simulink model "uGrid_1PH_hd_caso3"  (R2017a)
settings: Solver=VariableStepAuto  StartTime=0.0  StopTime=5  FixedStep=1e-6  MaxStep=1e-4  RelTol=1e-3
PreLoadFcn:
  | SimulinkInit
InitFcn:
  | SimulinkInit
StartFcn:
  | SimulinkInit
StopFcn:
  | EndingScript
undefined symbols (not defined in the file or in its folder): G, GF, Ion, J, K1, K2, K3, Lithium, P, Tao1, Tao2
libraries: powerlib x60, truetime x17, dsparch4 x12, powerlib_meascontrol x4, electricdrivelib x1, simulink x1
(part 1 of 2)
settings Model: SimulationMode=accelerator  Creator=erich  LastModifiedBy=carma

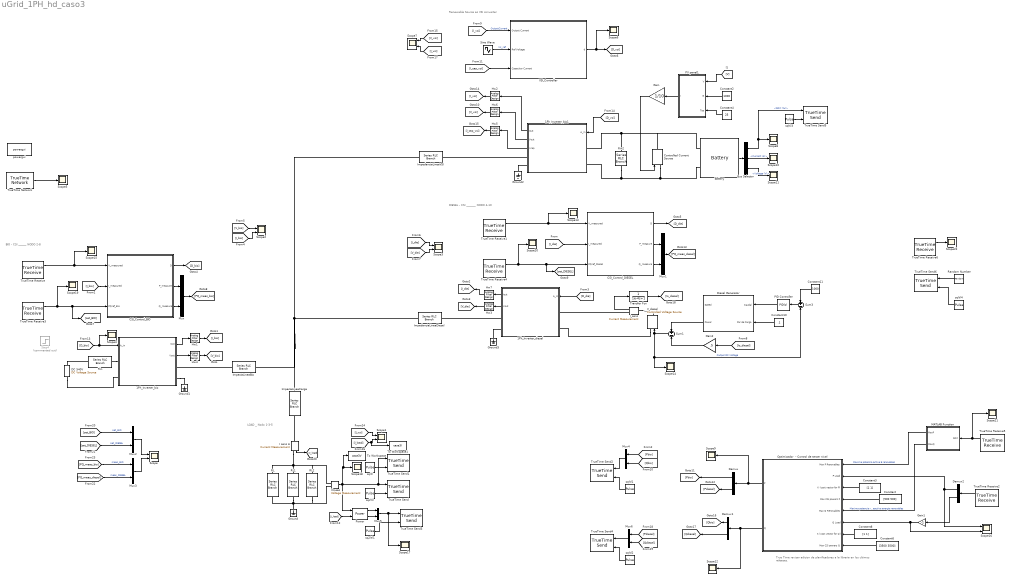
== system uGrid_1PH_hd_caso3 ==
  note: True Time revisar adicion de planificadores
      | a la libreria en los ultimos releases.
  note: Renewable Source as VSI converter
  note: LOAD _ Nodo 1-3-5
  note: BIO - CSI ______ NODO 2-8
  note: DIESEL - CSI _______ NODO 4-10
  1Ph_Inverter_bio : Subsystem  mask{st_time=4, f_sw=12000, samp_f=1e-6}
      mask prompts: st_time "Tiempo muerto (Start)"; f_sw "Switching frequency"; samp_f "samplig"
      mask Display:
      | port_label('input', 1, 'd', 'texmode', 'on')
      | 
      | port_label('lconn', 1, 'DC +')
      | port_label('lconn', 2, 'DC -')
      | 
      | 
      | port_label('rconn', 1, 'V_{out+}')
      | port_label('rconn', 2, 'B_{out-}')
      | 
      | 
      | port_label('output', 1, 'I_{out}', 'texmode', 'on')
      | port_label('output', 2, 'V_{out}', 'texmode', 'on')
      | 
      | plot([0.1 .9], [0.1 .9])
      | plot([0.2 .4], [.7 .7])
      | plot([0.2 .24], [.65 .65])
      | plot([0.28 .32], [.65 .65])
      | plot([0.36 .40], [.65 .65])
      | 
      | plot([.5:.01:.7], .25+sin(30*[.2:.01:.4])/10)
  1Ph_Inverter_bio1 : Subsystem  mask{st_time=1e-3, f_sw=12000, samp_f=1e-6}
      mask prompts: st_time "Tiempo muerto (Start)"; f_sw "Switching frequency"; samp_f "samplig"
      mask Display:
      | port_label('input', 1, 'd', 'texmode', 'on')
      | 
      | port_label('lconn', 1, 'DC +')
      | port_label('lconn', 2, 'DC -')
      | 
      | 
      | port_label('rconn', 1, 'V_{out+}')
      | port_label('rconn', 2, 'B_{out-}')
      | 
      | 
      | port_label('output', 1, 'I_{out}', 'texmode', 'on')
      | port_label('output', 2, 'V_{out}', 'texmode', 'on')
      | port_label('output', 3, 'I_{cap}', 'texmode', 'on')
      | 
      | plot([0.1 .9], [0.1 .9])
      | plot([0.2 .4], [.7 .7])
      | plot([0.2 .24], [.65 .65])
      | plot([0.28 .32], [.65 .65])
      | plot([0.36 .40], [.65 .65])
      | 
      | plot([.5:.01:.7], .25+sin(30*[.2:.01:.4])/10)
  1Ph_Inverter_diesel : Subsystem  mask{st_time=4, f_sw=12000, samp_f=1e-6}
      mask prompts: st_time "Tiempo muerto (Start)"; f_sw "Switching frequency"; samp_f "Sampling frequency"
      mask Display:
      | port_label('input', 1, 'd', 'texmode', 'on')
      | 
      | port_label('lconn', 1, 'DC +')
      | port_label('lconn', 2, 'DC -')
      | 
      | 
      | port_label('rconn', 1, 'V_{out+}')
      | port_label('rconn', 2, 'B_{out-}')
      | 
      | 
      | port_label('output', 1, 'I_{out}', 'texmode', 'on')
      | port_label('output', 2, 'V_{out}', 'texmode', 'on')
      | 
      | plot([0.1 .9], [0.1 .9])
      | plot([0.2 .4], [.7 .7])
      | plot([0.2 .24], [.65 .65])
      | plot([0.28 .32], [.65 .65])
      | plot([0.36 .40], [.65 .65])
      | 
      | plot([.5:.01:.7], .25+sin(30*[.2:.01:.4])/10)
  Battery : electricdrivelib/Extra Sources/Battery  BatType=Lithium-Ion  ShowTempParam=off  ThermalPreset=no  ShowAgeParam=off  NomV=1100  NomQ=.5  SOC=100  Batt_Tr=10e-3  PresetModel=off  MaxQ=1  MinV=825  FullV=1280.3859  Dis_rate=200  R=50e-3  Normal_OP=0.90435  expZone="[1188.4244    0.049130435]"  current=[6.5 13 32.5 50]  Units=Time  Tci=20  NomT=20  T2=-30  MaxQ2=4.8  FullV2=7.1  Normal_OP2=5.655  expZone2="[6.58           1]"  Rca=0.6  ti=2000  Dp=0  Neq0=0  Tsim=1e6  Ta1=25  Qeol=5.4*0.9  Reol=0.013333*1.2  Char_age=[2.3478, 3]  Dis_age=[2.3478, 10]  N1=1500  N2=10500  N3=1000  N4=1400  Ta2=45  N5=950
  Bus Selector : BusSelector  OutputSignals=SOC (%),Current (A),Voltage (V)
  CSI_Control_BIO : Subsystem
  CSI_Control_DIESEL : Subsystem
  Constant : Constant  Value=[500 500]
  Constant10 : Constant  Value=.1
  Constant11 : Constant  Value=1000
  Constant2 : Constant  Value=1000
  Constant3 : Constant  Value=[1 1]
  Constant4 : Constant  Value=25
  Constant6 : Constant  Value=[3500 3500]
  Constant8 : Constant  Value=[1 1]
  Controlled Current Source : powerlib/Electrical Sources/Controlled Current Source  Initialize=on  Source_Type=AC  Amplitude=0  Phase=0  Frequency=0  Measurements=None
  DC 540V : powerlib/Electrical Sources/DC Voltage Source  Amplitude=1000  Measurements=None
  Demux : Demux  Outputs=2
  Demux1 : Demux  Outputs=2
  Demux2 : Demux  Outputs=2
  Diesel Generator : Subsystem
  Gain : Gain  Gain=1/10
  Gain1 : Gain  Gain=-1
  Gain2 : Gain  Gain=.5
  Ground{,1..3} (4 alike) : powerlib/Elements/Ground  LConnTagsString=a
  Hw{1..7} (7 alike) : dsparch4/Analog Filter Design  method=Bessel  filttype=Lowpass  N=2  Wlo=7000*2*pi  Whi=80  Rp=2  Rs=80
  I sens A : powerlib/Measurements/Current Measurement  PhasorSimulation=off  OutputType=Complex  PSBequivalent=0
  I_sens : powerlib/Measurements/Current Measurement  PhasorSimulation=off  OutputType=Complex  PSBequivalent=0
  ImpeciaLineaBio : powerlib/Elements/Series RLC Branch  LConnTagsString=__new0  RConnTagsString=__new0  BranchType=RL  Resistance=.01  Inductance=1e-6  SetiL0=off  InitialCurrent=0  Capacitance=1e-6  Setx0=off  InitialVoltage=0  Measurements=None
  ImpeciaLineaCarga : powerlib/Elements/Series RLC Branch  LConnTagsString=__new0  RConnTagsString=__new0  BranchType=RL  Resistance=.01  Inductance=1e-6  SetiL0=off  InitialCurrent=0  Capacitance=1e-6  Setx0=off  InitialVoltage=0  Measurements=None
  ImpedanciaLineaDiesel : powerlib/Elements/Series RLC Branch  LConnTagsString=__new0  RConnTagsString=__new0  BranchType=RL  Resistance=.01  Inductance=1e-6  SetiL0=off  InitialCurrent=0  Capacitance=1e-6  Setx0=off  InitialVoltage=0  Measurements=None
  ImpedanciaLineaVSI : powerlib/Elements/Series RLC Branch  LConnTagsString=__new0  RConnTagsString=__new0  BranchType=R  Resistance=.01  Inductance=1e-6  SetiL0=off  InitialCurrent=0  Capacitance=1e-6  Setx0=off  InitialVoltage=0  Measurements=None
  MATLAB Function : MATLAB Function  TreatAsAtomicUnit=on
  Mux{,1..6} (7 alike) : Mux  Inputs=2
  Optimizador  - Control de tercer nivel : Subsystem
  PID Controller : simulink/Continuous/PID Controller  Controller=PID  TimeDomain=Continuous-time  SampleTime=-1  IntegratorMethod=Forward Euler  FilterMethod=Forward Euler  Form=Parallel  UseFilter=on  ControllerParametersSource=internal  P=0.000853612192208084  I=3.94394231511782e-05  D=0.00224356290205903  N=0.155980576752107  InitialConditionSource=internal  InitialConditionForIntegrator=0  InitialConditionForFilter=0  ExternalReset=none  LimitOutput=off  UpperSaturationLimit=inf  LowerSaturationLimit=-inf  LinearizeAsGain=on  AntiWindupMode=none  Kb=1  TrackingMode=off  Kt=1  PParamMin=[]  PParamMax=[]  IParamMin=[]  IParamMax=[]  DParamMin=[]  DParamMax=[]  NParamMin=[]  NParamMax=[]  KbParamMin=[]  KbParamMax=[]  KtParamMin=[]  KtParamMax=[]  POutMin=[]  POutMax=[]  IOutMin=[]  IOutMax=[]  DOutMin=[]  DOutMax=[]  NOutMin=[]  NOutMax=[]  KbOutMin=[]  KbOutMax=[]  KtOutMin=[]  KtOutMax=[]  IntegratorOutMin=[]  IntegratorOutMax=[]  FilterOutMin=[]  FilterOutMax=[]  SumOutMin=[]  SumOutMax=[]  SumI1OutMin=[]  SumI1OutMax=[]  SumI2OutMin=[]  SumI2OutMax=[]  SumI3OutMin=[]  SumI3OutMax=[]  SumDOutMin=[]  SumDOutMax=[]  SaturationOutMin=[]  SaturationOutMax=[]  IntegratorContinuousStateAttributes=''  IntegratorStateMustResolveToSignalObject=off  IntegratorRTWStateStorageClass=Auto  FilterContinuousStateAttributes=''  FilterStateMustResolveToSignalObject=off  FilterRTWStateStorageClass=Auto  DifferentiatorICPrevScaledInput=0  DifferentiatorOutMin=[]  DifferentiatorOutMax=[]  InitialConditionSetting=State (most efficient)
  PV panel1 : Subsystem
      mask Display: image('panel.jpg')
  Power : powerlib_meascontrol/Measurements/Power  Freq=60  Vinit=[1, 0]  Iinit=[1, 0]  Ts=0
      settings: SourceProductName=Simscape Power Systems
  RL : powerlib/Elements/Series RLC Branch  LConnTagsString=__new0  RConnTagsString=__new0  BranchType=R  Resistance=10  Inductance=500e-3  SetiL0=off  InitialCurrent=0  Capacitance=100e-6  Setx0=off  InitialVoltage=0  Measurements=None
  RL1 : powerlib/Elements/Series RLC Branch  LConnTagsString=__new0  RConnTagsString=__new0  BranchType=RL  Resistance=10  Inductance=5.2  SetiL0=off  InitialCurrent=0  Capacitance=100e-6  Setx0=off  InitialVoltage=0  Measurements=None
  RL2 : powerlib/Elements/Series RLC Branch  LConnTagsString=__new0  RConnTagsString=__new0  BranchType=C  Resistance=30  Inductance=500e-3  SetiL0=off  InitialCurrent=0  Capacitance=2000e-6  Setx0=off  InitialVoltage=0  Measurements=None
  Random Number : RandomNumber  SampleTime=0.1
  Rin : powerlib/Elements/Series RLC Branch  LConnTagsString=__new0  RConnTagsString=__new0  BranchType=R  Resistance=.001  Inductance=0  SetiL0=off  InitialCurrent=0  Capacitance=0  Setx0=off  InitialVoltage=0  Measurements=None
  Rin2 : powerlib/Elements/Series RLC Branch  LConnTagsString=__new0  RConnTagsString=__new0  BranchType=C  Resistance=.001  Inductance=0  SetiL0=off  InitialCurrent=0  Capacitance=1000e-6  Setx0=off  InitialVoltage=0  Measurements=None
  Scope{,1..3,7,16} (6 alike) : Scope  NumInputPorts=2
  Scope{4..6,8..15,17..22} (17 alike) : Scope
  Sine Wave : Sin  Amplitude=170  Frequency=2*pi*60  SampleTime=0
  Step4 : Step  Commented=on  Time=[2.3 2.3]  Before=[0 0]  After=[500 3500]  SampleTime=0
  Sum1 : Sum  Inputs=+-
  Sum3 : Sum  Inputs=+-
  To Workspace : ToWorkspace  VariableName=case3V  SaveFormat=Timeseries  SampleTime=1e-4
  To Workspace1 : ToWorkspace  VariableName=case3I  SaveFormat=Timeseries  SampleTime=1e-4
  Transfer Fcn : TransferFcn  Denominator=[1e-4 1]
  TrueTime Network : truetime/TrueTime Network  nwtype=CSMA/CD (Ethernet)  nwnbr=1  nnodes=14  rate=1000e7  minsize=100  lossprob=0  seed=0  bandwidths=[0.5 0.5]  slotsize=512  schedule=[1 1 2]  memsize=80000  buftype=Common buffer  overflow=Retransmit  dynSchedule=0  miniSlotSize=0  NIT=0  QSortMode=FIFO  sync=0  irtSchedule=0  nrtLength=0  nodeGraph=0  scheduleoutput=on
  TrueTime Receive : truetime/TrueTime Receive  nwnbr=1  receiver=2  outdim=1  triggeroutput=on  senderoutput=off  lengthoutput=off  priorityoutput=off  timestampoutput=off  signalpoweroutput=off  msgIDoutput=off
  TrueTime Receive1 : truetime/TrueTime Receive  nwnbr=1  receiver=4  outdim=1  triggeroutput=on  senderoutput=off  lengthoutput=off  priorityoutput=off  timestampoutput=off  signalpoweroutput=off  msgIDoutput=off
  TrueTime Receive2 : truetime/TrueTime Receive  nwnbr=1  receiver=6  outdim=2  triggeroutput=on  senderoutput=off  lengthoutput=off  priorityoutput=off  timestampoutput=off  signalpoweroutput=off  msgIDoutput=off
  TrueTime Receive3 : truetime/TrueTime Receive  nwnbr=1  receiver=8  outdim=2  triggeroutput=on  senderoutput=off  lengthoutput=off  priorityoutput=off  timestampoutput=off  signalpoweroutput=off  msgIDoutput=off
  TrueTime Receive4 : truetime/TrueTime Receive  nwnbr=1  receiver=10  outdim=2  triggeroutput=on  senderoutput=off  lengthoutput=off  priorityoutput=off  timestampoutput=off  signalpoweroutput=off  msgIDoutput=off
  TrueTime Receive5 : truetime/TrueTime Receive  nwnbr=1  receiver=12  outdim=1  triggeroutput=on  senderoutput=off  lengthoutput=off  priorityoutput=off  timestampoutput=off  signalpoweroutput=off  msgIDoutput=off
  TrueTime Receive6 : truetime/TrueTime Receive  nwnbr=1  receiver=14  outdim=1  triggeroutput=on  senderoutput=off  lengthoutput=off  priorityoutput=off  timestampoutput=off  signalpoweroutput=off  msgIDoutput=off
  TrueTime Send : truetime/TrueTime Send  trigger=falling  nwnbr=1  sender=3  indim=1  recsource=internal  receiver=4  lengthsource=internal  length=16  priosource=internal  prio=1  msgIDsource=internal  msgID=1  dynamicSegment=dynamic
  TrueTime Send1 : truetime/TrueTime Send  trigger=falling  nwnbr=1  sender=1  indim=1  recsource=internal  receiver=2  lengthsource=internal  length=16  priosource=internal  prio=1  msgIDsource=internal  msgID=0  dynamicSegment=dynamic
  TrueTime Send2 : truetime/TrueTime Send  trigger=falling  nwnbr=1  sender=7  indim=2  recsource=internal  receiver=8  lengthsource=internal  length=16  priosource=internal  prio=1  msgIDsource=internal  msgID=0  dynamicSegment=dynamic
  TrueTime Send3 : truetime/TrueTime Send  trigger=falling  nwnbr=1  sender=5  indim=2  recsource=internal  receiver=6  lengthsource=internal  length=16  priosource=internal  prio=1  msgIDsource=internal  msgID=0  dynamicSegment=dynamic
  TrueTime Send4 : truetime/TrueTime Send  trigger=falling  nwnbr=1  sender=9  indim=2  recsource=internal  receiver=10  lengthsource=internal  length=16  priosource=internal  prio=1  msgIDsource=internal  msgID=0  dynamicSegment=dynamic
  TrueTime Send5 : truetime/TrueTime Send  trigger=falling  nwnbr=1  sender=11  indim=1  recsource=internal  receiver=12  lengthsource=internal  length=16  priosource=internal  prio=1  msgIDsource=internal  msgID=0  dynamicSegment=dynamic
  TrueTime Send6 : truetime/TrueTime Send  trigger=falling  nwnbr=1  sender=13  indim=1  recsource=internal  receiver=14  lengthsource=internal  length=16384*16  priosource=internal  prio=1  msgIDsource=internal  msgID=0  dynamicSegment=dynamic
  VSI_Controller : Subsystem
  V_diesel : powerlib/Electrical Sources/Controlled Voltage Source  Initialize=on  Source_Type=AC  Amplitude=0  Phase=0  Frequency=0  Measurements=None
  Vmeas : powerlib/Measurements/Voltage Measurement  PhasorSimulation=off  OutputType=Complex  PSBequivalent=0
  powergui : powerlib/powergui  Priority=1  SimulationMode=Continuous  SampleTime=50e-6  frequency=60  Iterations=50  frequencyindice=0  Pbase=100e6  ErrMax=1e-4  UnitsV=kV  UnitsW=MW  buscounter=0  FunctionMessages=off  echomessages=off  EnableUseOfTLC=off  CurrentSourceSwitches=off  DisableSnubberDevices=off  DisableRonSwitches=off  DisableVfSwitches=off  DisplayEquations=off  SolverType=Tustin/Backward Euler (TBE)  Interpol=off  ExternalGateDelay=off  methode=off  Ts=100  x0status=blocks  SPID=on  SwTol=0  HookPort=off  RestoreLinks=warning  ResistiveCurrentMeasurement=off  Frange=[0:2:500]  Ylog=off  Xlog=on  ShowGrid=off  save=off  variable=ZData  structure=0  ZoomFFT=off  StartTime=0.0  cycles=1  DisplayStyle=1  fundamental=60  FreqAxis=off  MaxFrequency=1000  frequencyindicesteady=1  RmsSteady=1  display=off
  sq(t) : DiscretePulseGenerator  PulseType=Time based  Period=1e-4  PhaseDelay=1e-3
  sq(t)1 : DiscretePulseGenerator  PulseType=Time based  Period=.5  PhaseDelay=2e-3
  sq(t)2 : DiscretePulseGenerator  PulseType=Time based  Period=.5  PhaseDelay=3e-3
  sq(t)3 : DiscretePulseGenerator  PulseType=Time based  Period=.05  PhaseDelay=2e-3
  sq(t)4 : DiscretePulseGenerator  PulseType=Time based  Period=.5e-5  PhaseDelay=7e-3
  sq2(t) : DiscretePulseGenerator  PulseType=Time based  Period=1e-4  PhaseDelay=5e-3
  sq2(t)1 : DiscretePulseGenerator  PulseType=Time based  Period=.05
  wires:
  [D_bio] -> Scope4/1, 1Ph_Inverter_bio/1(A_in)
  [D_die] -> 1Ph_Inverter_diesel/1(A_in)
  [I_bio] -> Scope2/2
  [V_bio] -> Scope2/1
  [I_die] -> Scope3/1
  [V_die] -> Scope3/2
  1Ph_Inverter_bio/2(Vout) -> Hw4/1
  1Ph_Inverter_bio/1(Iout) -> Hw1/1
  Hw1/1 -> [I_bio]
  Hw4/1 -> [V_bio]
  1Ph_Inverter_diesel/1(Iout) -> Hw7/1
  Hw7/1 -> [I_die]
  Hw3/1 -> [V_die]
  1Ph_Inverter_diesel/2(Vout) -> Hw3/1
  I sens A/1 -> [I_load]
  CSI_Control_BIO/1(D) -> [D_bio]
  [I_bio] -> CSI_Control_BIO/2(I_measured)
  TrueTime Receive/1 -> Scope15/1, CSI_Control_BIO/1(V_measured)
  CSI_Control_DIESEL/1(D) -> [D_die]
  [I_die] -> CSI_Control_DIESEL/2(I_measured)
  TrueTime Receive1/1 -> Scope13/1, CSI_Control_DIESEL/1(V_measured)
  [I_vsi] -> Scope1/1
  [I_load] -> To Workspace1/1, Scope1/2
  Mux/1 -> [PQ_meas_bio]
  Mux1/1 -> [PQ_meas_diesel]
  [set_DIESEL] -> Mux2/2  "set_DIESEL"
  [set_BIO] -> Mux2/1  "set_BIO"
  Mux2/1 -> Scope/1
  Mux3/1 -> Scope/2
  [PQ_meas_diesel] -> Mux3/2  "meas_DIESEL"
  [PQ_meas_bio] -> Mux3/1  "meas_BIO"
  CSI_Control_BIO/2(P_measure) -> Mux/1
  CSI_Control_BIO/3(Q_measure) -> Mux/2
  CSI_Control_DIESEL/2(P_measure) -> Mux1/1
  CSI_Control_DIESEL/3(Q_measure) -> Mux1/2
  VSI_Controller/1(d) -> Scope6/1, [D_vsi]
  [I_vsi] -> VSI_Controller/1(Output Current)  "OutputCurrent"
  Sine Wave/1 -> VSI_Controller/2(Ref Voltage)  "Vc_ref"
  [I_cap_vsi] -> VSI_Controller/3(Capacitor Current)
  Hw5/1 -> [I_cap_vsi]
  1Ph_Inverter_bio1/3(I cap) -> Hw5/1
  1Ph_Inverter_bio1/2(Vout) -> Hw6/1
  1Ph_Inverter_bio1/1(Iout) -> Hw2/1
  [D_vsi] -> 1Ph_Inverter_bio1/1(A_in)
  Hw6/1 -> [V_vsi]
  Hw2/1 -> [I_vsi]
  [V_vsi] -> Scope7/1
  [I_vsi] -> Scope7/2
  Bus Selector/1 -> TrueTime Send5/1, Scope8/1  "<SOC (%)>"
  Bus Selector/3 -> Scope11/1  "<Voltage (V)>"
  Bus Selector/2 -> Scope10/1  "<Current (A)>"
  Battery/1 -> Bus Selector/1
  Constant2/1 -> PV panel1/2(G)
  [V] -> PV panel1/1(V)
  Constant4/1 -> PV panel1/3(Top)
  PV panel1/1(I) -> Gain/1
  Gain/1 -> Controlled Current Source/1
  TrueTime Receive4/1 -> Scope20/1, [set_DIESEL], CSI_Control_DIESEL/3(PQref_Diesel)
  Vmeas/1 -> To Workspace/1, Scope18/1, Power/1, TrueTime Send1/1, TrueTime Send/1
  sq2(t)/1 -> TrueTime Send/2
  TrueTime Network/1 -> Scope5/1
  MATLAB Function/1(MaxP) -> Optimizador  - Control de tercer nivel/1(Max P Renovables)  "Maxima potencia activa E renovables"
  Demux2/1 -> Optimizador  - Control de tercer nivel/2(P Load), Scope16/1
  Constant3/1 -> Optimizador  - Control de tercer nivel/3(K (cost vector for P))
  Constant/1 -> Optimizador  - Control de tercer nivel/4(Max CSI powers P)
  MATLAB Function/2(MaxQ) -> Optimizador  - Control de tercer nivel/5(Max Q Renovables)  "Maxima potencia reactiva energia renovables"
  Demux2/2 -> Gain1/1
  Constant8/1 -> Optimizador  - Control de tercer nivel/7(K (cost vector for Q))
  Constant6/1 -> Optimizador  - Control de tercer nivel/8(Max CSI powers Q)
  Optimizador  - Control de tercer nivel/2(Q) -> Demux1/1, Scope12/1
  Optimizador  - Control de tercer nivel/1(P) -> Demux/1, Scope9/1
  Demux/1 -> [Pbio]
  Demux/2 -> [Pdiesel]
  Demux1/2 -> [Qdiesel]
  Demux1/1 -> [Qbio]
  Constant10/1 -> Diesel Generator/2(Par de Carga)
  sq(t)/1 -> TrueTime Send1/2
  Transfer Fcn/1 -> [Io_diesel]
  I_sens/1 -> Transfer Fcn/1
  Gain2/1 -> Sum1/2
  [Io_diesel] -> Gain2/1
  Constant11/1 -> Sum3/1
  Sum3/1 -> PID Controller/1
  Sum1/1 -> Scope14/1, Sum3/2, V_diesel/1  "Output DC Voltage"
  PID Controller/1 -> Diesel Generator/1(Caudal)
  Diesel Generator/2(Power) -> Sum1/1
  sq(t)1/1 -> TrueTime Send2/2
  [Qbio] -> Mux4/2
  [Pbio] -> Mux4/1
  Mux4/1 -> TrueTime Send2/1
  [I_load] -> Power/2
  Power/1 -> Mux5/1
  Power/2 -> Mux5/2
  Mux5/1 -> Scope17/1, TrueTime Send3/1
  sq2(t)1/1 -> TrueTime Send3/2
  TrueTime Receive2/1 -> Demux2/1
  [Pdiesel] -> Mux6/1
  [Qdiesel] -> Mux6/2
  Mux6/1 -> TrueTime Send4/1
  sq(t)2/1 -> TrueTime Send4/2
  TrueTime Receive3/1 -> Scope19/1, [set_BIO], CSI_Control_BIO/3(PQref_Bio)
  Gain1/1 -> Scope16/2, Optimizador  - Control de tercer nivel/6(Q Load)
  sq(t)3/1 -> TrueTime Send5/2
  TrueTime Receive5/1 -> Scope21/1, MATLAB Function/1(SOC)
  sq(t)4/1 -> TrueTime Send6/2
  Random Number/1 -> TrueTime Send6/1
  TrueTime Receive6/1 -> Scope22/1
  connections:
  RL/LConn1 -- RL2/LConn1 -- Vmeas/LConn1 -- I sens A/RConn1 -- RL1/LConn1
  Ground/LConn1 -- Vmeas/LConn2 -- RL2/RConn1 -- RL1/RConn1 -- RL/RConn1
  1Ph_Inverter_bio/RConn2 -- Ground1/LConn1
  DC 540V/LConn1 -- 1Ph_Inverter_bio/LConn2
  Rin/RConn1 -- 1Ph_Inverter_bio/LConn1
  1Ph_Inverter_diesel/RConn2 -- Ground3/LConn1
  1Ph_Inverter_diesel/RConn1 -- ImpedanciaLineaDiesel/RConn1
  DC 540V/RConn1 -- Rin/LConn1
  1Ph_Inverter_bio1/RConn2 -- Ground2/LConn1
  Rin2/RConn1 -- 1Ph_Inverter_bio1/LConn2 -- Controlled Current Source/LConn1 -- Battery/LConn2
  Rin2/LConn1 -- Controlled Current Source/RConn1 -- Battery/LConn1 -- 1Ph_Inverter_bio1/LConn1
  V_diesel/LConn1 -- 1Ph_Inverter_diesel/LConn2
  I_sens/LConn1 -- V_diesel/RConn1
  I_sens/RConn1 -- 1Ph_Inverter_diesel/LConn1
  ImpeciaLineaBio/LConn1 -- 1Ph_Inverter_bio/RConn1
  ImpedanciaLineaDiesel/LConn1 -- ImpedanciaLineaVSI/LConn1 -- ImpeciaLineaCarga/LConn1 -- ImpeciaLineaBio/RConn1
  1Ph_Inverter_bio1/RConn1 -- ImpedanciaLineaVSI/RConn1
  I sens A/LConn1 -- ImpeciaLineaCarga/RConn1

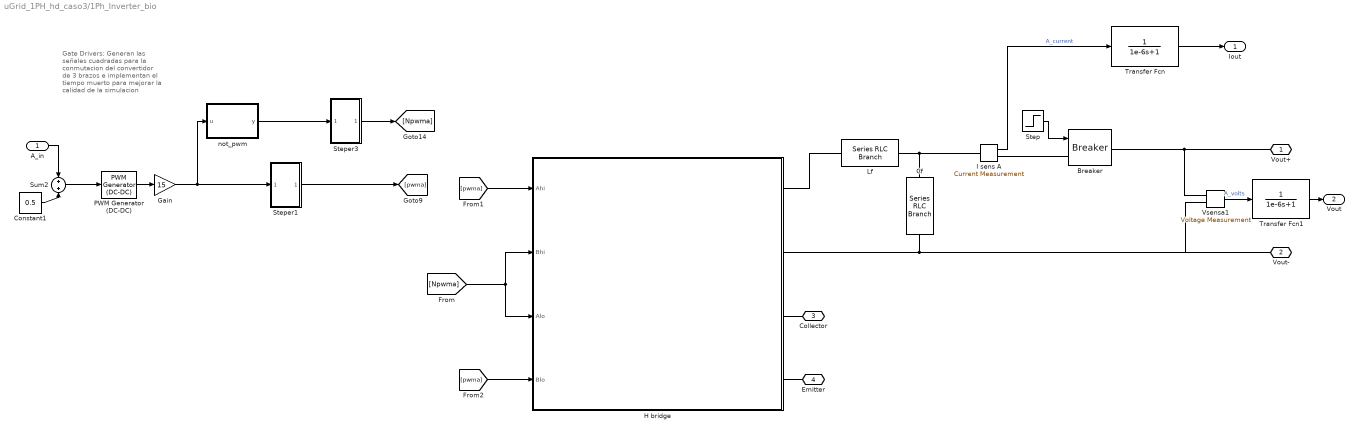
== system uGrid_1PH_hd_caso3/1Ph_Inverter_bio ==
  note: Gate Drivers: Generan las señales cuadradas para
      | la conmutacion del convertidor de 3 brazos e implementan el
      | tiempo muerto para mejorar la calidad de la simulacion
  A_in : Inport
  Breaker : powerlib/Elements/Breaker  InitialState=0  SwitchingTimes="[1/60  5/60]"  External=on  BreakerResistance=0.01  SnubberResistance=1e6  SnubberCapacitance=inf  Measurements=None  MoreParameters=on  NoBreakLoop=off
      settings: SourceProductName=Simscape Power Systems
  Cf : powerlib/Elements/Series RLC Branch  LConnTagsString=__new0  RConnTagsString=__new0  BranchType=C  Resistance=1  Inductance=1e-3  SetiL0=off  InitialCurrent=0  Capacitance=22e-6  Setx0=off  InitialVoltage=0  Measurements=None
  Constant1 : Constant  Value=0.5
  Gain : Gain  Gain=15
  H bridge : Subsystem
      mask Display:
      | port_label('input', 1, '\fontsize{12} Ahi', 'texmode', 'on')
      | port_label('input', 2, '\fontsize{12} Alo', 'texmode', 'on')
      | port_label('input', 3, '\fontsize{12} Bhi', 'texmode', 'on')
      | port_label('input', 4, '\fontsize{12} Blo', 'texmode', 'on')
      | 
      | 
      | port_label('rconn', 1, '\fontsize{12} V_{out} +', 'texmode', 'on')
      | port_label('rconn', 2, '\fontsize{12} V_{out} -', 'texmode', 'on')
      | 
      | port_label('rconn', 3, '\fontsize{12} Collector', 'texmode', 'on')
      | port_label('rconn', 4, '\fontsize{12} Emitter', 'texmode', 'on')
      | 
      | lvx = [.1 .1];
      | lvy = [.1 .2];
      | lhx = [.1 .2];
      | lhy = [.1 .1];
      | 
      | 
      | % se dibujan los interruptores de la izquierda
      | plot(lvx+.07, lvy*.8+.028+.1)
      | plot(lvx+.1, lvy+.1)
      | plot(lhx*.5+.15, lhy+.1)
      | plot(lhx*.5+.15, lhy+.2)
      | plot(lhx*.5+.07, lhy+.15)
      | 
      | d=0.5;
      | 
      | plot(lvx+.07, lvy*.8+.028+.1+d)
      | plot(lvx+.1, lvy+.1+d)
      | plot(lhx*.5+.15, lhy+.1+d)
      | plot(lhx*.5+.15, lhy+.2+d)
      | plot(lhx*.5+.07, lhy+.15+d)
      | 
      | 
      | % se dibujan los interruptores del medio
      | h=.3;
      | 
      | %plot(lvx+.07+h, lvy*.8+.028+.1)
      | %plot(lvx+.1+h, lvy+.1)
      | %plot(lhx*.5+.15+h, lhy+.1)
      | %plot(lhx*.5+.15+h, lhy+.2)
      | %plot(lhx*.5+.07+h, lhy+.15)
      | 
      | %plot(lvx+.07+h, lvy*.8+.028+.1+d)
      | %plot(lvx+.1+h, lvy+.1+d)
      | %plot(lhx*.5+.15+h, lhy+.1+d)
      | %plot(lhx*.5+.15+h, lhy+.2+d)
      | %plot(lhx*.5+.07+h, lhy+.15+d)
      | 
      | % se dibujan los interruptores de la derecha
      | h=.6
      | 
      | plot(lvx+.07+h, lvy*.8+.028+.1)
      | plot(lvx+.1+h, lvy+.1)
      | plot(lhx*.5+.15+h, lhy+.1)
      | plot(lhx*.5+.15+h, lhy+.2)
      | plot(lhx*.5+.07+h, lhy+.15)
      | 
      | plot(lvx+.07+h, lvy*.8+.028+.1+d)
      | plot(lvx+.1+h, lvy+.1+d)
      | plot(lhx*.5+.15+h, lhy+.1+d)
      | plot(lhx*.5+.15+h, lhy+.2+d)
      | plot(lhx*.5+.07+h, lhy+.15+d)
      | 
      | 
      | % se conectan los interruptores.
      | plot(lvx+.15, lvy*4-.1)
      | %plot(lvx+.15+.3, lvy*4-.1)
      | plot(lvx+.15+.6, lvy*4-.1)
      | 
      | 
      | plot(lvx+.15, lvy+.7)
      | %plot(lvx+.15+.3, lvy+.7)
      | plot(lvx+.15+.6, lvy+.7)
      | 
      | plot(lvx+.15, lvy)
      | %plot(lvx+.15+.3, lvy)
      | plot(lvx+.15+.6, lvy)
      | 
      | plot(lhx*6-.35, lhy)
      | plot(lhx*6-.35, lhy+.8)
      | 
      | % raul esteban alzate 313 515 86 11
  I sens A : powerlib/Measurements/Current Measurement  PhasorSimulation=off  OutputType=Complex  PSBequivalent=0
  Lf : powerlib/Elements/Series RLC Branch  LConnTagsString=__new0  RConnTagsString=__new0  BranchType=RL  Resistance=.1  Inductance=40e-3  SetiL0=off  InitialCurrent=0  Capacitance=1e-6  Setx0=off  InitialVoltage=0  Measurements=None
  PWM Generator (DC-DC) : powerlib_meascontrol/Pulse & Signal Generators/PWM Generator (DC-DC)  Fsw=f_sw  Ts=samp_f
  Step : Step  Time=st_time  SampleTime=0
  Steper1 : Subsystem
  Steper3 : Subsystem
  Sum2 : Sum
  Transfer Fcn : TransferFcn  Denominator=[1e-6 1]
  Transfer Fcn1 : TransferFcn  Denominator=[1e-6 1]
  Vsensa1 : powerlib/Measurements/Voltage Measurement  PhasorSimulation=off  OutputType=Complex  PSBequivalent=0
  not_pwm : MATLAB Function  TreatAsAtomicUnit=on
  Vout+ : PMIOPort  Port=1  Side=Right
  Vout- : PMIOPort  Port=2  Side=Right
  Collector : PMIOPort  Port=3  Side=Left
  Emitter : PMIOPort  Port=4  Side=Left
  Iout : Outport
  Vout : Outport  Port=2
  wires:
  not_pwm/1(y) -> Steper3/1(In1)
  Sum2/1 -> PWM Generator (DC-DC)/1
  PWM Generator (DC-DC)/1 -> Gain/1
  Constant1/1 -> Sum2/2
  A_in/1 -> Sum2/1
  Steper1/1(Out1) -> [pwma]
  Steper3/1(Out1) -> [Npwma]
  Gain/1 -> Steper1/1(In1), not_pwm/1(u)
  [pwma] -> H bridge/1(Ahi)
  [Npwma] -> H bridge/2(Bhi), H bridge/3(Alo)
  [pwma] -> H bridge/4(Blo)
  I sens A/1 -> Transfer Fcn/1  "A_current"
  Vsensa1/1 -> Transfer Fcn1/1  "A_volts"
  Transfer Fcn/1 -> Iout/1
  Transfer Fcn1/1 -> Vout/1
  Step/1 -> Breaker/1
  connections:
  H bridge/RConn3 -- Collector/RConn1
  H bridge/RConn4 -- Emitter/RConn1
  Lf/LConn1 -- H bridge/RConn1
  H bridge/RConn2 -- Vsensa1/LConn2 -- Vout-/RConn1 -- Cf/RConn1
  Breaker/LConn1 -- I sens A/RConn1
  Breaker/RConn1 -- Vout+/RConn1 -- Vsensa1/LConn1
  Cf/LConn1 -- I sens A/LConn1 -- Lf/RConn1

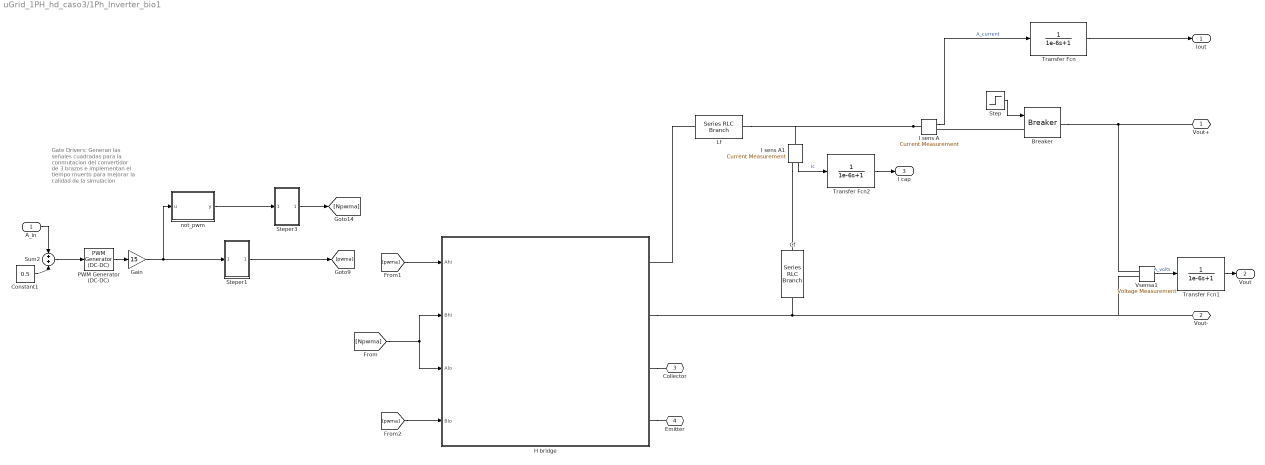
== system uGrid_1PH_hd_caso3/1Ph_Inverter_bio1 ==
  note: Gate Drivers: Generan las señales cuadradas para
      | la conmutacion del convertidor de 3 brazos e implementan el
      | tiempo muerto para mejorar la calidad de la simulacion
  A_in : Inport
  Breaker : powerlib/Elements/Breaker  InitialState=0  SwitchingTimes="[1/60  5/60]"  External=on  BreakerResistance=0.01  SnubberResistance=1e6  SnubberCapacitance=inf  Measurements=None  MoreParameters=on  NoBreakLoop=off
      settings: SourceProductName=Simscape Power Systems
  Cf : powerlib/Elements/Series RLC Branch  LConnTagsString=__new0  RConnTagsString=__new0  BranchType=C  Resistance=1  Inductance=1e-3  SetiL0=off  InitialCurrent=0  Capacitance=610e-6  Setx0=off  InitialVoltage=0  Measurements=None
  Constant1 : Constant  Value=0.5
  Gain : Gain  Gain=15
  H bridge : Subsystem
      mask Display:
      | port_label('input', 1, '\fontsize{12} Ahi', 'texmode', 'on')
      | port_label('input', 2, '\fontsize{12} Alo', 'texmode', 'on')
      | port_label('input', 3, '\fontsize{12} Bhi', 'texmode', 'on')
      | port_label('input', 4, '\fontsize{12} Blo', 'texmode', 'on')
      | 
      | 
      | port_label('rconn', 1, '\fontsize{12} V_{out} +', 'texmode', 'on')
      | port_label('rconn', 2, '\fontsize{12} V_{out} -', 'texmode', 'on')
      | 
      | port_label('rconn', 3, '\fontsize{12} Collector', 'texmode', 'on')
      | port_label('rconn', 4, '\fontsize{12} Emitter', 'texmode', 'on')
      | 
      | lvx = [.1 .1];
      | lvy = [.1 .2];
      | lhx = [.1 .2];
      | lhy = [.1 .1];
      | 
      | 
      | % se dibujan los interruptores de la izquierda
      | plot(lvx+.07, lvy*.8+.028+.1)
      | plot(lvx+.1, lvy+.1)
      | plot(lhx*.5+.15, lhy+.1)
      | plot(lhx*.5+.15, lhy+.2)
      | plot(lhx*.5+.07, lhy+.15)
      | 
      | d=0.5;
      | 
      | plot(lvx+.07, lvy*.8+.028+.1+d)
      | plot(lvx+.1, lvy+.1+d)
      | plot(lhx*.5+.15, lhy+.1+d)
      | plot(lhx*.5+.15, lhy+.2+d)
      | plot(lhx*.5+.07, lhy+.15+d)
      | 
      | 
      | % se dibujan los interruptores del medio
      | h=.3;
      | 
      | %plot(lvx+.07+h, lvy*.8+.028+.1)
      | %plot(lvx+.1+h, lvy+.1)
      | %plot(lhx*.5+.15+h, lhy+.1)
      | %plot(lhx*.5+.15+h, lhy+.2)
      | %plot(lhx*.5+.07+h, lhy+.15)
      | 
      | %plot(lvx+.07+h, lvy*.8+.028+.1+d)
      | %plot(lvx+.1+h, lvy+.1+d)
      | %plot(lhx*.5+.15+h, lhy+.1+d)
      | %plot(lhx*.5+.15+h, lhy+.2+d)
      | %plot(lhx*.5+.07+h, lhy+.15+d)
      | 
      | % se dibujan los interruptores de la derecha
      | h=.6
      | 
      | plot(lvx+.07+h, lvy*.8+.028+.1)
      | plot(lvx+.1+h, lvy+.1)
      | plot(lhx*.5+.15+h, lhy+.1)
      | plot(lhx*.5+.15+h, lhy+.2)
      | plot(lhx*.5+.07+h, lhy+.15)
      | 
      | plot(lvx+.07+h, lvy*.8+.028+.1+d)
      | plot(lvx+.1+h, lvy+.1+d)
      | plot(lhx*.5+.15+h, lhy+.1+d)
      | plot(lhx*.5+.15+h, lhy+.2+d)
      | plot(lhx*.5+.07+h, lhy+.15+d)
      | 
      | 
      | % se conectan los interruptores.
      | plot(lvx+.15, lvy*4-.1)
      | %plot(lvx+.15+.3, lvy*4-.1)
      | plot(lvx+.15+.6, lvy*4-.1)
      | 
      | 
      | plot(lvx+.15, lvy+.7)
      | %plot(lvx+.15+.3, lvy+.7)
      | plot(lvx+.15+.6, lvy+.7)
      | 
      | plot(lvx+.15, lvy)
      | %plot(lvx+.15+.3, lvy)
      | plot(lvx+.15+.6, lvy)
      | 
      | plot(lhx*6-.35, lhy)
      | plot(lhx*6-.35, lhy+.8)
      | 
      | % raul esteban alzate 313 515 86 11
  I sens A : powerlib/Measurements/Current Measurement  PhasorSimulation=off  OutputType=Complex  PSBequivalent=0
  I sens A1 : powerlib/Measurements/Current Measurement  PhasorSimulation=off  OutputType=Complex  PSBequivalent=0
  Lf : powerlib/Elements/Series RLC Branch  LConnTagsString=__new0  RConnTagsString=__new0  BranchType=RL  Resistance=1e-3  Inductance=5e-3  SetiL0=off  InitialCurrent=0  Capacitance=1e-6  Setx0=off  InitialVoltage=0  Measurements=None
  PWM Generator (DC-DC) : powerlib_meascontrol/Pulse & Signal Generators/PWM Generator (DC-DC)  Fsw=f_sw  Ts=samp_f
  Step : Step  Time=st_time  SampleTime=0
  Steper1 : Subsystem
  Steper3 : Subsystem
  Sum2 : Sum
  Transfer Fcn : TransferFcn  Denominator=[1e-6 1]
  Transfer Fcn1 : TransferFcn  Denominator=[1e-6 1]
  Transfer Fcn2 : TransferFcn  Denominator=[1e-6 1]
  Vsensa1 : powerlib/Measurements/Voltage Measurement  PhasorSimulation=off  OutputType=Complex  PSBequivalent=0
  not_pwm : MATLAB Function  TreatAsAtomicUnit=on
  Vout+ : PMIOPort  Port=1  Side=Right
  Vout- : PMIOPort  Port=2  Side=Right
  Collector : PMIOPort  Port=3  Side=Left
  Emitter : PMIOPort  Port=4  Side=Left
  Iout : Outport
  Vout : Outport  Port=2
  I cap : Outport  Port=3
  wires:
  not_pwm/1(y) -> Steper3/1(In1)
  Sum2/1 -> PWM Generator (DC-DC)/1
  PWM Generator (DC-DC)/1 -> Gain/1
  Constant1/1 -> Sum2/2
  A_in/1 -> Sum2/1
  Steper1/1(Out1) -> [pwma]
  Steper3/1(Out1) -> [Npwma]
  Gain/1 -> Steper1/1(In1), not_pwm/1(u)
  [pwma] -> H bridge/1(Ahi)
  [Npwma] -> H bridge/2(Bhi), H bridge/3(Alo)
  [pwma] -> H bridge/4(Blo)
  I sens A/1 -> Transfer Fcn/1  "A_current"
  Vsensa1/1 -> Transfer Fcn1/1  "A_volts"
  Transfer Fcn/1 -> Iout/1
  Transfer Fcn1/1 -> Vout/1
  Step/1 -> Breaker/1
  Transfer Fcn2/1 -> I cap/1
  I sens A1/1 -> Transfer Fcn2/1  "Ic"
  connections:
  H bridge/RConn3 -- Collector/RConn1
  H bridge/RConn4 -- Emitter/RConn1
  Lf/LConn1 -- H bridge/RConn1
  H bridge/RConn2 -- Vout-/RConn1 -- Vsensa1/LConn2 -- Cf/RConn1
  Breaker/LConn1 -- I sens A/RConn1
  Breaker/RConn1 -- Vsensa1/LConn1 -- Vout+/RConn1
  I sens A/LConn1 -- Lf/RConn1 -- I sens A1/LConn1
  I sens A1/RConn1 -- Cf/LConn1

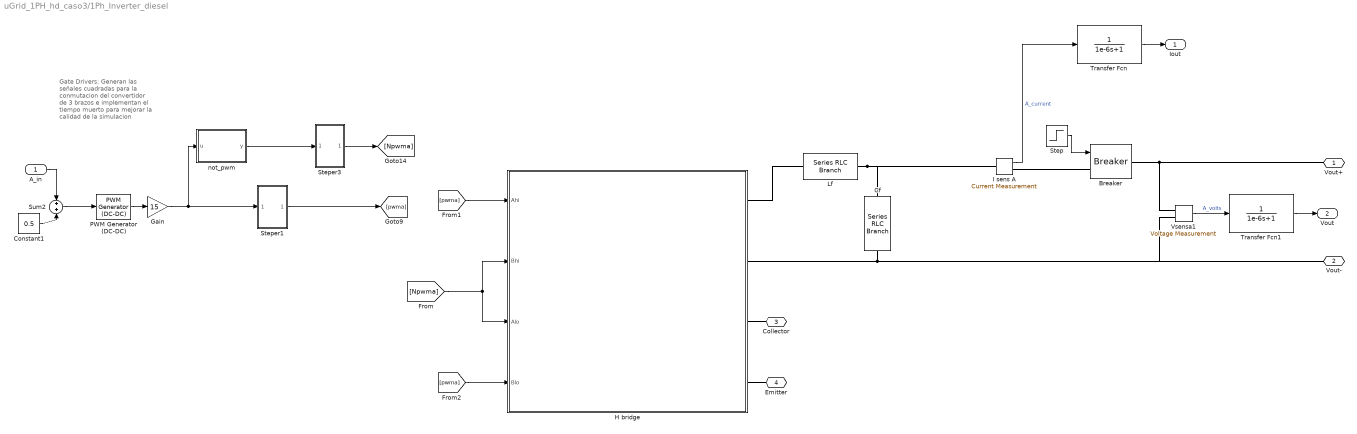
== system uGrid_1PH_hd_caso3/1Ph_Inverter_diesel ==
  note: Gate Drivers: Generan las señales cuadradas para
      | la conmutacion del convertidor de 3 brazos e implementan el
      | tiempo muerto para mejorar la calidad de la simulacion
  A_in : Inport
  Breaker : powerlib/Elements/Breaker  InitialState=0  SwitchingTimes="[1/60  5/60]"  External=on  BreakerResistance=0.01  SnubberResistance=1e6  SnubberCapacitance=inf  Measurements=None  MoreParameters=on  NoBreakLoop=off
      settings: SourceProductName=Simscape Power Systems
  Cf : powerlib/Elements/Series RLC Branch  LConnTagsString=__new0  RConnTagsString=__new0  BranchType=C  Resistance=1  Inductance=1e-3  SetiL0=off  InitialCurrent=0  Capacitance=22e-6  Setx0=off  InitialVoltage=0  Measurements=None
  Constant1 : Constant  Value=0.5
  Gain : Gain  Gain=15
  H bridge : Subsystem
      mask Display:
      | port_label('input', 1, '\fontsize{12} Ahi', 'texmode', 'on')
      | port_label('input', 2, '\fontsize{12} Alo', 'texmode', 'on')
      | port_label('input', 3, '\fontsize{12} Bhi', 'texmode', 'on')
      | port_label('input', 4, '\fontsize{12} Blo', 'texmode', 'on')
      | 
      | 
      | port_label('rconn', 1, '\fontsize{12} V_{out} +', 'texmode', 'on')
      | port_label('rconn', 2, '\fontsize{12} V_{out} -', 'texmode', 'on')
      | 
      | port_label('rconn', 3, '\fontsize{12} Collector', 'texmode', 'on')
      | port_label('rconn', 4, '\fontsize{12} Emitter', 'texmode', 'on')
      | 
      | lvx = [.1 .1];
      | lvy = [.1 .2];
      | lhx = [.1 .2];
      | lhy = [.1 .1];
      | 
      | 
      | % se dibujan los interruptores de la izquierda
      | plot(lvx+.07, lvy*.8+.028+.1)
      | plot(lvx+.1, lvy+.1)
      | plot(lhx*.5+.15, lhy+.1)
      | plot(lhx*.5+.15, lhy+.2)
      | plot(lhx*.5+.07, lhy+.15)
      | 
      | d=0.5;
      | 
      | plot(lvx+.07, lvy*.8+.028+.1+d)
      | plot(lvx+.1, lvy+.1+d)
      | plot(lhx*.5+.15, lhy+.1+d)
      | plot(lhx*.5+.15, lhy+.2+d)
      | plot(lhx*.5+.07, lhy+.15+d)
      | 
      | 
      | % se dibujan los interruptores del medio
      | h=.3;
      | 
      | %plot(lvx+.07+h, lvy*.8+.028+.1)
      | %plot(lvx+.1+h, lvy+.1)
      | %plot(lhx*.5+.15+h, lhy+.1)
      | %plot(lhx*.5+.15+h, lhy+.2)
      | %plot(lhx*.5+.07+h, lhy+.15)
      | 
      | %plot(lvx+.07+h, lvy*.8+.028+.1+d)
      | %plot(lvx+.1+h, lvy+.1+d)
      | %plot(lhx*.5+.15+h, lhy+.1+d)
      | %plot(lhx*.5+.15+h, lhy+.2+d)
      | %plot(lhx*.5+.07+h, lhy+.15+d)
      | 
      | % se dibujan los interruptores de la derecha
      | h=.6
      | 
      | plot(lvx+.07+h, lvy*.8+.028+.1)
      | plot(lvx+.1+h, lvy+.1)
      | plot(lhx*.5+.15+h, lhy+.1)
      | plot(lhx*.5+.15+h, lhy+.2)
      | plot(lhx*.5+.07+h, lhy+.15)
      | 
      | plot(lvx+.07+h, lvy*.8+.028+.1+d)
      | plot(lvx+.1+h, lvy+.1+d)
      | plot(lhx*.5+.15+h, lhy+.1+d)
      | plot(lhx*.5+.15+h, lhy+.2+d)
      | plot(lhx*.5+.07+h, lhy+.15+d)
      | 
      | 
      | % se conectan los interruptores.
      | plot(lvx+.15, lvy*4-.1)
      | %plot(lvx+.15+.3, lvy*4-.1)
      | plot(lvx+.15+.6, lvy*4-.1)
      | 
      | 
      | plot(lvx+.15, lvy+.7)
      | %plot(lvx+.15+.3, lvy+.7)
      | plot(lvx+.15+.6, lvy+.7)
      | 
      | plot(lvx+.15, lvy)
      | %plot(lvx+.15+.3, lvy)
      | plot(lvx+.15+.6, lvy)
      | 
      | plot(lhx*6-.35, lhy)
      | plot(lhx*6-.35, lhy+.8)
      | 
      | % raul esteban alzate 313 515 86 11
  I sens A : powerlib/Measurements/Current Measurement  PhasorSimulation=off  OutputType=Complex  PSBequivalent=0
  Lf : powerlib/Elements/Series RLC Branch  LConnTagsString=__new0  RConnTagsString=__new0  BranchType=RL  Resistance=.1  Inductance=30e-3  SetiL0=off  InitialCurrent=0  Capacitance=1e-6  Setx0=off  InitialVoltage=0  Measurements=None
  PWM Generator (DC-DC) : powerlib_meascontrol/Pulse & Signal Generators/PWM Generator (DC-DC)  Fsw=f_sw  Ts=samp_f
  Step : Step  Time=st_time  SampleTime=0
  Steper1 : Subsystem
  Steper3 : Subsystem
  Sum2 : Sum
  Transfer Fcn : TransferFcn  Denominator=[1e-6 1]
  Transfer Fcn1 : TransferFcn  Denominator=[1e-6 1]
  Vsensa1 : powerlib/Measurements/Voltage Measurement  PhasorSimulation=off  OutputType=Complex  PSBequivalent=0
  not_pwm : MATLAB Function  TreatAsAtomicUnit=on
  Vout+ : PMIOPort  Port=1  Side=Right
  Vout- : PMIOPort  Port=2  Side=Right
  Collector : PMIOPort  Port=3  Side=Left
  Emitter : PMIOPort  Port=4  Side=Left
  Iout : Outport
  Vout : Outport  Port=2
  wires:
  Vsensa1/1 -> Transfer Fcn1/1  "A_volts"
  I sens A/1 -> Transfer Fcn/1  "A_current"
  [pwma] -> H bridge/4(Blo)
  [Npwma] -> H bridge/3(Alo), H bridge/2(Bhi)
  [pwma] -> H bridge/1(Ahi)
  Gain/1 -> not_pwm/1(u), Steper1/1(In1)
  Steper3/1(Out1) -> [Npwma]
  Steper1/1(Out1) -> [pwma]
  A_in/1 -> Sum2/1
  Constant1/1 -> Sum2/2
  PWM Generator (DC-DC)/1 -> Gain/1
  Sum2/1 -> PWM Generator (DC-DC)/1
  not_pwm/1(y) -> Steper3/1(In1)
  Transfer Fcn/1 -> Iout/1
  Transfer Fcn1/1 -> Vout/1
  Step/1 -> Breaker/1
  connections:
  Cf/RConn1 -- Vsensa1/LConn2 -- Vout-/RConn1 -- H bridge/RConn2
  Lf/LConn1 -- H bridge/RConn1
  H bridge/RConn4 -- Emitter/RConn1
  H bridge/RConn3 -- Collector/RConn1
  Breaker/LConn1 -- I sens A/RConn1
  Breaker/RConn1 -- Vsensa1/LConn1 -- Vout+/RConn1
  Lf/RConn1 -- I sens A/LConn1 -- Cf/LConn1

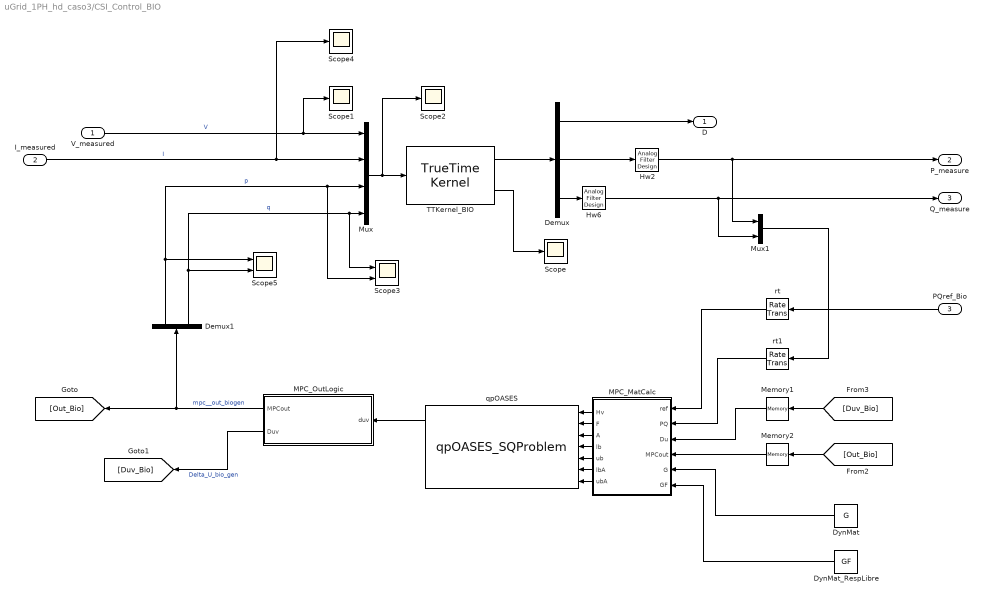
== system uGrid_1PH_hd_caso3/CSI_Control_BIO ==
  V_measured : Inport
  I_measured : Inport  Port=2
  PQref_Bio : Inport  Port=3
  Demux : Demux  Outputs=3
  Demux1 : Demux  Outputs=2
  DynMat : Constant  Value=G
  DynMat_RespLibre : Constant  Value=GF
  Hw2 : dsparch4/Analog Filter Design  method=Bessel  filttype=Lowpass  N=4  Wlo=30*2*pi  Whi=80  Rp=2  Rs=80
  Hw6 : dsparch4/Analog Filter Design  method=Bessel  filttype=Lowpass  N=4  Wlo=30*2*pi  Whi=80  Rp=2  Rs=80
  MPC_MatCalc : MATLAB Function  TreatAsAtomicUnit=on  SystemSampleTime=1e-3
      settings: MinAlgLoopOccurrences=on
  MPC_OutLogic : MATLAB Function  TreatAsAtomicUnit=on
      settings: MinAlgLoopOccurrences=on
  Memory1 : Memory
  Memory2 : Memory
  Mux : Mux
  Mux1 : Mux  Inputs=2
  Scope{,1..2,4} (4 alike) : Scope
  Scope3 : Scope  NumInputPorts=2
  Scope5 : Scope  NumInputPorts=2
  TTKernel_BIO : truetime/TrueTime Kernel  sfun=BIO_init  args=1  ninputsoutputs=[4 3]  ntriggers=0  trigtype=falling  nwnodenbr=[]  clockoffsetdrift=[0 0]  schedoutput=on  battery=off  poweroutput=off
  qpOASES : S-Function  FunctionName=qpOASES_SQProblem  SFunctionDeploymentMode=off  EnableBusSupport=off
  rt : RateTransition  X0=[0 0]  OutPortSampleTime=1e-3
  rt1 : RateTransition  X0=[0 0]  OutPortSampleTime=1e-3
  D : Outport
  P_measure : Outport  Port=2
  Q_measure : Outport  Port=3
  wires:
  TTKernel_BIO/1 -> Demux/1
  Demux/3 -> Hw6/1
  Demux/2 -> Hw2/1
  Demux/1 -> D/1
  TTKernel_BIO/2 -> Scope/1
  Mux/1 -> Scope2/1, TTKernel_BIO/1
  V_measured/1 -> Scope1/1, Mux/1  "V"
  I_measured/1 -> Scope4/1, Mux/2  "I"
  Demux1/1 -> Scope5/1, Scope3/2, Mux/3  "p"
  Demux1/2 -> Scope5/2, Scope3/1, Mux/4  "q"
  Hw6/1 -> Mux1/2, Q_measure/1
  Hw2/1 -> Mux1/1, P_measure/1
  PQref_Bio/1 -> rt/1
  MPC_MatCalc/5(ub) -> qpOASES/5
  qpOASES/1 -> MPC_OutLogic/1(duv)
  [Duv_Bio] -> Memory1/1
  MPC_OutLogic/1(MPCout) -> [Out_Bio], Demux1/1  "mpc__out_biogen"
  MPC_MatCalc/7(ubA) -> qpOASES/7
  MPC_MatCalc/1(Hv) -> qpOASES/1
  MPC_MatCalc/2(F) -> qpOASES/2
  Memory2/1 -> MPC_MatCalc/4(MPCout)
  MPC_OutLogic/2(Duv) -> [Duv_Bio]  "Delta_U_bio_gen"
  DynMat/1 -> MPC_MatCalc/5(G)
  MPC_MatCalc/3(A) -> qpOASES/3
  MPC_MatCalc/6(lbA) -> qpOASES/6
  Memory1/1 -> MPC_MatCalc/3(Du)
  DynMat_RespLibre/1 -> MPC_MatCalc/6(GF)
  rt/1 -> MPC_MatCalc/1(ref)
  [Out_Bio] -> Memory2/1
  MPC_MatCalc/4(lb) -> qpOASES/4
  rt1/1 -> MPC_MatCalc/2(PQ)
  Mux1/1 -> rt1/1

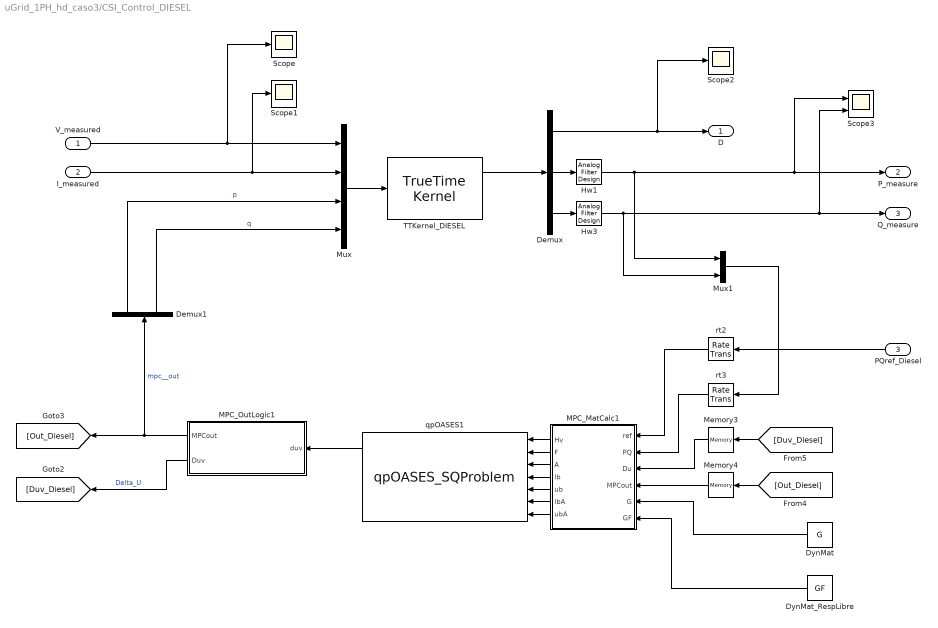
== system uGrid_1PH_hd_caso3/CSI_Control_DIESEL ==
  V_measured : Inport
  I_measured : Inport  Port=2
  PQref_Diesel : Inport  Port=3
  Demux : Demux  Outputs=3
  Demux1 : Demux  Outputs=2
  DynMat : Constant  Value=G
  DynMat_RespLibre : Constant  Value=GF
  Hw1 : dsparch4/Analog Filter Design  method=Bessel  filttype=Lowpass  N=4  Wlo=30*2*pi  Whi=80  Rp=2  Rs=80
  Hw3 : dsparch4/Analog Filter Design  method=Bessel  filttype=Lowpass  N=4  Wlo=30*2*pi  Whi=80  Rp=2  Rs=80
  MPC_MatCalc1 : MATLAB Function  TreatAsAtomicUnit=on  SystemSampleTime=1e-3
      settings: MinAlgLoopOccurrences=on
  MPC_OutLogic1 : MATLAB Function  TreatAsAtomicUnit=on
      settings: MinAlgLoopOccurrences=on
  Memory3 : Memory
  Memory4 : Memory
  Mux : Mux
  Mux1 : Mux  Inputs=2
  Scope : Scope
  Scope1 : Scope
  Scope2 : Scope
  Scope3 : Scope  NumInputPorts=2
  TTKernel_DIESEL : truetime/TrueTime Kernel  sfun=DIESEL_init  args=[]  ninputsoutputs=[4 3]  ntriggers=0  trigtype=falling  nwnodenbr=[]  clockoffsetdrift=[0 0]  schedoutput=on  battery=off  poweroutput=off
  qpOASES1 : S-Function  FunctionName=qpOASES_SQProblem  SFunctionDeploymentMode=off  EnableBusSupport=off
  rt2 : RateTransition  X0=[0 0]  OutPortSampleTime=1e-3
  rt3 : RateTransition  X0=[0 0]  OutPortSampleTime=1e-3
  D : Outport
  P_measure : Outport  Port=2
  Q_measure : Outport  Port=3
  wires:
  Mux/1 -> TTKernel_DIESEL/1
  Demux/3 -> Hw3/1
  Demux/2 -> Hw1/1
  TTKernel_DIESEL/1 -> Demux/1
  Demux/1 -> Scope2/1, D/1
  Hw1/1 -> Mux1/1, Scope3/1, P_measure/1
  Hw3/1 -> Mux1/2, Scope3/2, Q_measure/1
  Demux1/1 -> Mux/3  "p"
  Demux1/2 -> Mux/4  "q"
  I_measured/1 -> Scope1/1, Mux/2
  V_measured/1 -> Scope/1, Mux/1
  [Out_Diesel] -> Memory4/1
  MPC_MatCalc1/3(A) -> qpOASES1/3
  MPC_OutLogic1/1(MPCout) -> Demux1/1, [Out_Diesel]  "mpc__out"
  qpOASES1/1 -> MPC_OutLogic1/1(duv)
  DynMat/1 -> MPC_MatCalc1/5(G)
  rt3/1 -> MPC_MatCalc1/2(PQ)
  MPC_MatCalc1/7(ubA) -> qpOASES1/7
  MPC_MatCalc1/1(Hv) -> qpOASES1/1
  Memory3/1 -> MPC_MatCalc1/3(Du)
  rt2/1 -> MPC_MatCalc1/1(ref)
  MPC_OutLogic1/2(Duv) -> [Duv_Diesel]  "Delta_U"
  [Duv_Diesel] -> Memory3/1
  MPC_MatCalc1/5(ub) -> qpOASES1/5
  MPC_MatCalc1/2(F) -> qpOASES1/2
  DynMat_RespLibre/1 -> MPC_MatCalc1/6(GF)
  MPC_MatCalc1/4(lb) -> qpOASES1/4
  Mux1/1 -> rt3/1
  PQref_Diesel/1 -> rt2/1
  Memory4/1 -> MPC_MatCalc1/4(MPCout)
  MPC_MatCalc1/6(lbA) -> qpOASES1/6

== system uGrid_1PH_hd_caso3/Diesel Generator ==
  Caudal : Inport
  Par de Carga : Inport  Port=2
  " 1" : Gain  Gain=K1
  " Generador1" : Gain  Gain=1/2
  Actuador1 : TransferFcn  Numerator=[K3*K2]  Denominator=[Tao2 1]
  Dinámica en el eje1 : TransferFcn  Numerator=[(J*P)]  Denominator=[1 (J*P)]
  Gain1 : Gain  Gain=12000
  Motor de Combustión1 : TransportDelay  DelayTime=Tao1
  Sum2 : Sum  Inputs=|+-
  Speed : Outport
  Power : Outport  Port=2
  wires:
  " 1"/1 -> Motor de Combustión1/1
  " Generador1"/1 -> Gain1/1
  Motor de Combustión1/1 -> Sum2/1
  Actuador1/1 -> " 1"/1
  Dinámica en el eje1/1 -> Speed/1, " Generador1"/1  "Velocidad"
  Sum2/1 -> Dinámica en el eje1/1
  Caudal/1 -> Actuador1/1
  Par de Carga/1 -> Sum2/2
  Gain1/1 -> Power/1

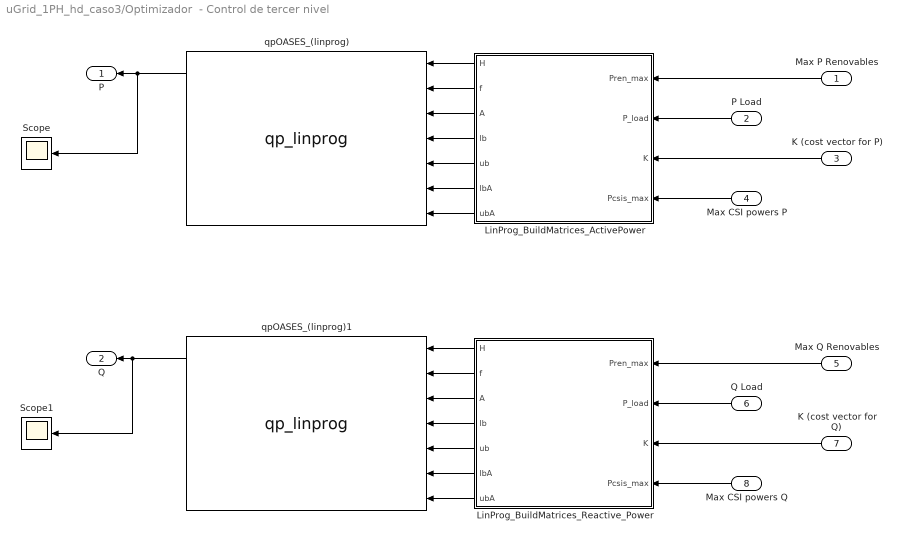
== system uGrid_1PH_hd_caso3/Optimizador  - Control de tercer nivel ==
  Max P Renovables : Inport
  P Load : Inport  Port=2
  K (cost vector for P) : Inport  Port=3
  Max CSI powers P : Inport  Port=4
  Max Q Renovables : Inport  Port=5
  Q Load : Inport  Port=6
  K (cost vector for Q) : Inport  Port=7
  Max CSI powers Q : Inport  Port=8
  LinProg_BuildMatrices_ActivePower : MATLAB Function  TreatAsAtomicUnit=on
  LinProg_BuildMatrices_Reactive_Power : MATLAB Function  TreatAsAtomicUnit=on
  Scope : Scope
  Scope1 : Scope
  qpOASES_(linprog) : S-Function  FunctionName=qp_linprog  SFunctionDeploymentMode=off  EnableBusSupport=off
  qpOASES_(linprog)1 : S-Function  FunctionName=qp_linprog  SFunctionDeploymentMode=off  EnableBusSupport=off
  P : Outport
  Q : Outport  Port=2
  wires:
  Max CSI powers P/1 -> LinProg_BuildMatrices_ActivePower/4(Pcsis_max)
  Max P Renovables/1 -> LinProg_BuildMatrices_ActivePower/1(Pren_max)
  LinProg_BuildMatrices_ActivePower/6(lbA) -> qpOASES_(linprog)/6
  LinProg_BuildMatrices_ActivePower/5(ub) -> qpOASES_(linprog)/5
  LinProg_BuildMatrices_ActivePower/7(ubA) -> qpOASES_(linprog)/7
  LinProg_BuildMatrices_ActivePower/2(f) -> qpOASES_(linprog)/2
  LinProg_BuildMatrices_ActivePower/4(lb) -> qpOASES_(linprog)/4
  LinProg_BuildMatrices_ActivePower/1(H) -> qpOASES_(linprog)/1
  K (cost vector for P)/1 -> LinProg_BuildMatrices_ActivePower/3(K)
  P Load/1 -> LinProg_BuildMatrices_ActivePower/2(P_load)
  LinProg_BuildMatrices_ActivePower/3(A) -> qpOASES_(linprog)/3
  LinProg_BuildMatrices_Reactive_Power/1(H) -> qpOASES_(linprog)1/1
  LinProg_BuildMatrices_Reactive_Power/5(ub) -> qpOASES_(linprog)1/5
  LinProg_BuildMatrices_Reactive_Power/3(A) -> qpOASES_(linprog)1/3
  LinProg_BuildMatrices_Reactive_Power/4(lb) -> qpOASES_(linprog)1/4
  LinProg_BuildMatrices_Reactive_Power/6(lbA) -> qpOASES_(linprog)1/6
  LinProg_BuildMatrices_Reactive_Power/2(f) -> qpOASES_(linprog)1/2
  LinProg_BuildMatrices_Reactive_Power/7(ubA) -> qpOASES_(linprog)1/7
  qpOASES_(linprog)/1 -> Scope/1, P/1
  qpOASES_(linprog)1/1 -> Scope1/1, Q/1
  Q Load/1 -> LinProg_BuildMatrices_Reactive_Power/2(P_load)
  K (cost vector for Q)/1 -> LinProg_BuildMatrices_Reactive_Power/3(K)
  Max Q Renovables/1 -> LinProg_BuildMatrices_Reactive_Power/1(Pren_max)
  Max CSI powers Q/1 -> LinProg_BuildMatrices_Reactive_Power/4(Pcsis_max)

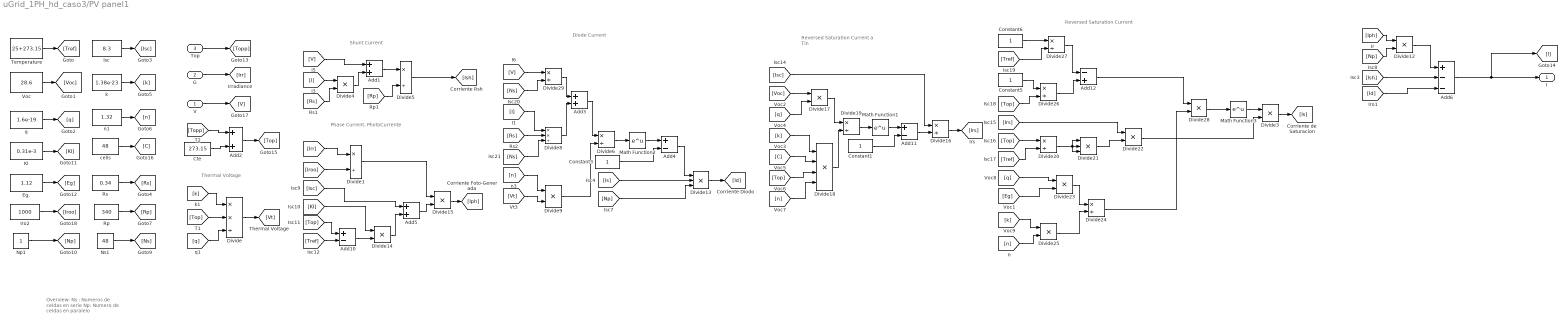
== system uGrid_1PH_hd_caso3/PV panel1 ==
  note: Overview:
      | Ns : Numeros de celdas en serie
      | Np: Numero de celdas en paralelo
  note: Thermal Voltage
  note: Shunt Current
  note: Phase Current- PhotoCurrente
  note: Diode Current
  note: Reversed Saturation Current a Tin
  note: Reversed Saturation Current
  V : Inport
  G : Inport  Port=2
  Top : Inport  Port=3
  Add{1..3,5} (4 alike) : Sum
  Add10 : Sum  Inputs=+-
  Add11 : Sum  Inputs=+-
  Add12 : Sum  Inputs=-+
  Add4 : Sum  Inputs=+-
  Add6 : Sum  Inputs=+--
  Constant{1,3,5..6} (4 alike) : Constant
  Cte : Constant  Value=273.15
  Divide : Product  Inputs=**/
  Divide{1,5..6,16,19..20,24,26..27,29} (10 alike) : Product  Inputs=*/
  Divide{3..4,9,12,14..15,17,22..23,25,28} (11 alike) : Product  Inputs=**
  Divide13 : Product  Inputs=***
  Divide18 : Product  Inputs=****
  Divide21 : Product  Inputs=***
  Divide8 : Product  Inputs=**/
  Eg. : Constant  Value=1.12
  Iro2 : Constant  Value=1000
  Isc : Constant  Value=8.3
  KI : Constant  Value=0.31e-3
  Math Function1 : Math  SaturateOnIntegerOverflow=on
  Math Function2 : Math  SaturateOnIntegerOverflow=on
  Math Function3 : Math  SaturateOnIntegerOverflow=on
  Np1 : Constant
  Ns1 : Constant  Value=48
  Rp : Constant  Value=340
  Rs : Constant  Value=0.34
  Temperature : Constant  Value=25+273.15
  Voc : Constant  Value=28.6
  cells : Constant  Value=48
  k : Constant  Value=1.38e-23
  n1 : Constant  Value=1.32
  q : Constant  Value=1.6e-19
  I : Outport
  wires:
  Temperature/1 -> [Tref]
  Voc/1 -> [Voc]
  q/1 -> [q]
  Isc/1 -> [Isc]
  k/1 -> [k]
  n1/1 -> [n]
  [k] -> Divide/1
  [Top] -> Divide/2
  [q] -> Divide/3
  Divide/1 -> [Vt]
  Divide3/1 -> [Is]
  [Ish] -> Add6/2
  Add6/1 -> I/1, [I]
  [I] -> Divide8/1
  [Rs] -> Divide8/2
  Divide8/1 -> Add3/2
  [n] -> Divide9/1
  [Vt] -> Divide9/2
  Divide9/1 -> Divide6/2
  Add3/1 -> Divide6/1
  Divide6/1 -> Math Function2/1
  Math Function2/1 -> Add4/1
  Add4/1 -> Divide13/1
  [Is] -> Divide13/2
  Divide13/1 -> [Id]
  Divide4/1 -> Add1/2
  Add1/1 -> Divide5/1
  [Rp] -> Divide5/2
  Divide5/1 -> [Ish]
  [Rs] -> Divide4/2
  [I] -> Divide4/1
  KI/1 -> [KI]
  Eg./1 -> [Eg]
  [V] -> Add1/1
  [Np] -> Divide13/3
  [Iph] -> Divide12/1
  [Np] -> Divide12/2
  Divide12/1 -> Add6/1
  [Isc] -> Add5/1
  [Top] -> Add10/1
  [Tref] -> Add10/2
  Add10/1 -> Divide14/2
  [KI] -> Divide14/1
  [Voc] -> Divide17/1
  [q] -> Divide17/2
  [k] -> Divide18/1
  [C] -> Divide18/2
  [Top] -> Divide18/3
  [n] -> Divide18/4
  Divide17/1 -> Divide19/1
  Divide18/1 -> Divide19/2
  Divide19/1 -> Math Function1/1
  Constant1/1 -> Add11/2
  Math Function1/1 -> Add11/1
  Add11/1 -> Divide16/2
  Divide16/1 -> [Irs]
  [Tref] -> Divide20/2
  [Top] -> Divide20/1
  Divide20/1 -> Divide21/2, Divide21/1, Divide21/3
  Divide21/1 -> Divide22/2
  [Irs] -> Divide22/1
  [q] -> Divide23/1
  Divide23/1 -> Divide24/1
  [k] -> Divide25/1
  [n] -> Divide25/2
  Divide25/1 -> Divide24/2
  Constant5/1 -> Divide26/1
  [Top] -> Divide26/2
  Constant6/1 -> Divide27/1
  [Tref] -> Divide27/2
  Divide27/1 -> Add12/1
  Divide26/1 -> Add12/2
  Add12/1 -> Divide28/1
  Divide24/1 -> Divide28/2
  Divide28/1 -> Math Function3/1
  Divide29/1 -> Add3/1
  [Ns] -> Divide29/2
  [V] -> Divide29/1
  [Ns] -> Divide8/3
  Divide14/1 -> Add5/2
  Add5/1 -> Divide15/2
  Divide15/1 -> [Iph]
  V/1 -> [V]
  G/1 -> [Irr]
  Top/1 -> [Topp]
  cells/1 -> [C]
  [Id] -> Add6/3
  Cte/1 -> Add2/2
  Add2/1 -> [Top]
  [Topp] -> Add2/1
  [Irr] -> Divide1/1
  [Iroo] -> Divide1/2
  Divide1/1 -> Divide15/1
  Iro2/1 -> [Iroo]
  Rs/1 -> [Rs]
  Rp/1 -> [Rp]
  Ns1/1 -> [Ns]
  Np1/1 -> [Np]
  Constant3/1 -> Add4/2
  [Isc] -> Divide16/1
  Math Function3/1 -> Divide3/1
  Divide22/1 -> Divide3/2
  [Eg] -> Divide23/2

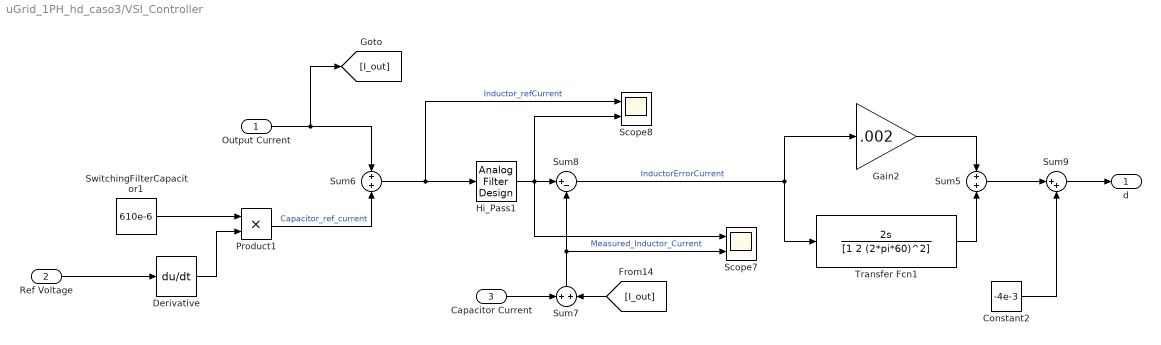
== system uGrid_1PH_hd_caso3/VSI_Controller ==
  Output Current : Inport
  Ref Voltage : Inport  Port=2
  Capacitor Current : Inport  Port=3
  Constant2 : Constant  Value=-4e-3
  Derivative : Derivative  CoefficientInTFapproximation=1e-3
  Gain2 : Gain  Gain=.002
  Hi_Pass1 : dsparch4/Analog Filter Design  method=Bessel  filttype=Highpass  N=1  Wlo=1*2*pi  Whi=80  Rp=2  Rs=40
  Product1 : Product
  Scope7 : Scope  NumInputPorts=2
  Scope8 : Scope  NumInputPorts=2
  Sum5 : Sum  Inputs=+|+
  Sum6 : Sum  Inputs=+|+
  Sum7 : Sum  Inputs=+|+
  Sum8 : Sum  Inputs=|+-
  Sum9 : Sum  Inputs=|++
  SwitchingFilterCapacitor1 : Constant  Value=610e-6
  Transfer Fcn1 : TransferFcn  Numerator=[2 0]  Denominator=[1 2 (2*pi*60)^2]
  d : Outport
  wires:
  Derivative/1 -> Product1/2
  Sum6/1 -> Hi_Pass1/1, Scope8/1  "Inductor_refCurrent"
  Sum8/1 -> Transfer Fcn1/1, Gain2/1  "InductorErrorCurrent"
  Ref Voltage/1 -> Derivative/1
  Constant2/1 -> Sum9/2
  Capacitor Current/1 -> Sum7/1
  Transfer Fcn1/1 -> Sum5/2
  Output Current/1 -> Sum6/1, [I_out]
  [I_out] -> Sum7/2
  Gain2/1 -> Sum5/1
  SwitchingFilterCapacitor1/1 -> Product1/1
  Hi_Pass1/1 -> Scope8/2, Sum8/1, Scope7/1
  Product1/1 -> Sum6/2  "Capacitor_ref_current"
  Sum9/1 -> d/1
  Sum5/1 -> Sum9/1
  Sum7/1 -> Scope7/2, Sum8/2  "Measured_Inductor_Current"
